simulink model "Model"  (R2018b)
settings: Solver=FixedStepAuto  StartTime=0.0  StopTime=10000  RelTol=1e-3
values from neighbouring files (symbols this model uses):
  Cb = 1000    [workspace.m]
  Ch = 2700    [workspace.m]
  Cw = 4200    [workspace.m]
  Cwym = 2700    [workspace.m]
  Fzcomax = 150    [workspace.m]
  Kext = 15000    [workspace.m]
  Kh = 12000    [workspace.m]
  Kw = 250000    [workspace.m]
  Mb = 20000    [workspace.m]
  Mco = 3000    [workspace.m]
  Mh = 3000    [workspace.m]
  Mm = 3000    [workspace.m]
  ro = 1000    [workspace.m]
  T0 = 5    [workspace.m]
  TrSP = 15    [workspace.m]
libraries: simulink x2
settings Model: Creator=Konrad  LastModifiedBy=Konrad

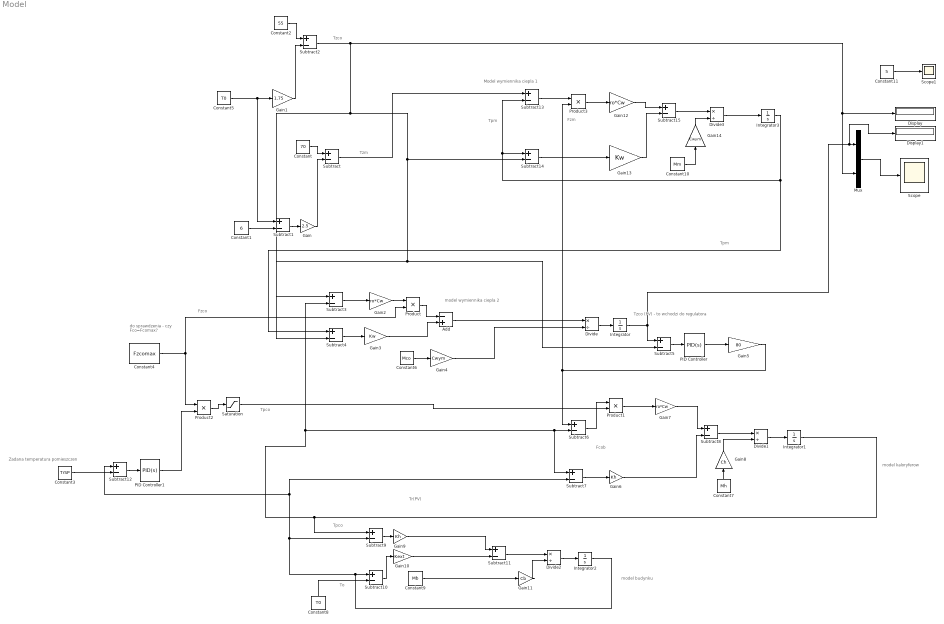
== system Model ==
  note: Model wymiennika ciepla 1
  note: do sprawdzenia
      | - czy Fco=Fcomax?
  note: model budynku
  note: Fcob
  note: Tr(PV)
  note: model kaloryferow
  note: model wymiennika ciepla 2
  note: Tzco (PV) - to wchodzi do regulatora
  note: Fzco
  note: Tpco
  note: Tpm
  note: Tzco
  note: Tzm
  note: Tpco
  note: To
  note: Zadana temperatura pomieszczen
  note: Tpm
  note: Fzm
  Add : Sum  Inputs=-+
  Constant : Constant  Value=70
  Constant1 : Constant  Value=6
  Constant10 : Constant  Value=Mm
  Constant11 : Constant  Value=5
  Constant2 : Constant  Value=55
  Constant3 : Constant  Value=TrSP
  Constant4 : Constant  Value=Fzcomax
  Constant5 : Constant  Value=T0
  Constant6 : Constant  Value=Mco
  Constant7 : Constant  Value=Mh
  Constant8 : Constant  Value=T0
  Constant9 : Constant  Value=Mb
  Display : Display
  Display1 : Display
  Divide{,1..3} (4 alike) : Product  Inputs=*/
  Gain : Gain  Gain=2.5
  Gain1 : Gain  Gain=1.75
  Gain10 : Gain  Gain=Kext
  Gain11 : Gain  Gain=Cb
  Gain12 : Gain  Gain=ro*Cw
  Gain13 : Gain  Gain=Kw
  Gain14 : Gain  Gain=Cwym
  Gain2 : Gain  Gain=ro*Cw
  Gain3 : Gain  Gain=Kw
  Gain4 : Gain  Gain=Cwym
  Gain5 : Gain  Gain=80
  Gain6 : Gain  Gain=Kh
  Gain7 : Gain  Gain=ro*Cw
  Gain8 : Gain  Gain=Ch
  Gain9 : Gain  Gain=Kh
  Integrator{,1..3} (4 alike) : Integrator
  Mux : Mux  Inputs=2
  PID Controller : simulink/Continuous/PID Controller  Controller=PID  Form=Parallel  TimeDomain=Continuous-time  SampleTime=-1  IntegratorMethod=Forward Euler  FilterMethod=Forward Euler  ControllerParametersSource=internal  P=0.01  I=0.1  D=0  UseFilter=on  N=100  TunerSelectOption=Transfer Function Based (PID Tuner App)  InitialConditionSource=internal  InitialConditionForIntegrator=0  InitialConditionForFilter=0  DifferentiatorICPrevScaledInput=0  ExternalReset=none  TrackingMode=off  Kt=1  LimitOutput=on  UpperSaturationLimit=1  LowerSaturationLimit=0  LinearizeAsGain=on  AntiWindupMode=none  Kb=1  POutMin=[]  POutMax=[]  IOutMin=[]  IOutMax=[]  DOutMin=[]  DOutMax=[]  NOutMin=[]  NOutMax=[]  SumOutMin=[]  SumOutMax=[]  SaturationOutMin=[]  SaturationOutMax=[]  PParamMin=[]  PParamMax=[]  IParamMin=[]  IParamMax=[]  DParamMin=[]  DParamMax=[]  NParamMin=[]  NParamMax=[]  KbParamMin=[]  KbParamMax=[]  KtParamMin=[]  KtParamMax=[]  KbOutMin=[]  KbOutMax=[]  KtOutMin=[]  KtOutMax=[]  IntegratorOutMin=[]  IntegratorOutMax=[]  FilterOutMin=[]  FilterOutMax=[]  SumI1OutMin=[]  SumI1OutMax=[]  SumI2OutMin=[]  SumI2OutMax=[]  SumI3OutMin=[]  SumI3OutMax=[]  SumI4OutMin=[]  SumI4OutMax=[]  SumDOutMin=[]  SumDOutMax=[]  DifferentiatorOutMin=[]  DifferentiatorOutMax=[]  FilterDiffOutCoefMin=[]  FilterDiffOutCoefMax=[]  ReciprocalOutMin=[]  ReciprocalOutMax=[]  SumDenOutMin=[]  SumDenOutMax=[]  SumNumOutMin=[]  SumNumOutMax=[]  DivideOutMin=[]  DivideOutMax=[]  IntegratorContinuousStateAttributes=''  IntegratorStateMustResolveToSignalObject=off  IntegratorRTWStateStorageClass=Auto  FilterContinuousStateAttributes=''  FilterStateMustResolveToSignalObject=off  FilterRTWStateStorageClass=Auto  ParallelPVariant=InternalParameters  IdealPVariant=Disabled  IVariant=InternalParameters  DVariant=InternalParameters  IntegratorVariant=Continuous  SatVariant=Enabled  AWVariant=Passthrough  PCopyVariant=Disabled  TRVariant=Disabled  FdbkBlocksVariant=Forward  IdealPFdbkVariant=Disabled  SatFdbkVariant=Disabled  DerivativeFilterVariant=ContFilter  NVariant=InternalParameters  NCopyVariant=Disabled  FilterICVariant=InternalICsFilter  IntegratorICVariant=InternalICs  ExternalResetVariant=Disabled  TRSumVariant=Passthrough  SumFdbkVariant=Disabled  SumVariant=Sum_PID
  PID Controller1 : simulink/Continuous/PID Controller  Controller=PID  Form=Parallel  TimeDomain=Continuous-time  SampleTime=-1  IntegratorMethod=Forward Euler  FilterMethod=Forward Euler  ControllerParametersSource=internal  P=0.01  I=0.1  D=0  UseFilter=on  N=100  TunerSelectOption=Transfer Function Based (PID Tuner App)  InitialConditionSource=internal  InitialConditionForIntegrator=0  InitialConditionForFilter=0  DifferentiatorICPrevScaledInput=0  ExternalReset=none  TrackingMode=off  Kt=1  LimitOutput=on  UpperSaturationLimit=1  LowerSaturationLimit=0  LinearizeAsGain=on  AntiWindupMode=none  Kb=1  POutMin=[]  POutMax=[]  IOutMin=[]  IOutMax=[]  DOutMin=[]  DOutMax=[]  NOutMin=[]  NOutMax=[]  SumOutMin=[]  SumOutMax=[]  SaturationOutMin=[]  SaturationOutMax=[]  PParamMin=[]  PParamMax=[]  IParamMin=[]  IParamMax=[]  DParamMin=[]  DParamMax=[]  NParamMin=[]  NParamMax=[]  KbParamMin=[]  KbParamMax=[]  KtParamMin=[]  KtParamMax=[]  KbOutMin=[]  KbOutMax=[]  KtOutMin=[]  KtOutMax=[]  IntegratorOutMin=[]  IntegratorOutMax=[]  FilterOutMin=[]  FilterOutMax=[]  SumI1OutMin=[]  SumI1OutMax=[]  SumI2OutMin=[]  SumI2OutMax=[]  SumI3OutMin=[]  SumI3OutMax=[]  SumI4OutMin=[]  SumI4OutMax=[]  SumDOutMin=[]  SumDOutMax=[]  DifferentiatorOutMin=[]  DifferentiatorOutMax=[]  FilterDiffOutCoefMin=[]  FilterDiffOutCoefMax=[]  ReciprocalOutMin=[]  ReciprocalOutMax=[]  SumDenOutMin=[]  SumDenOutMax=[]  SumNumOutMin=[]  SumNumOutMax=[]  DivideOutMin=[]  DivideOutMax=[]  IntegratorContinuousStateAttributes=''  IntegratorStateMustResolveToSignalObject=off  IntegratorRTWStateStorageClass=Auto  FilterContinuousStateAttributes=''  FilterStateMustResolveToSignalObject=off  FilterRTWStateStorageClass=Auto  ParallelPVariant=InternalParameters  IdealPVariant=Disabled  IVariant=InternalParameters  DVariant=InternalParameters  IntegratorVariant=Continuous  SatVariant=Enabled  AWVariant=Passthrough  PCopyVariant=Disabled  TRVariant=Disabled  FdbkBlocksVariant=Forward  IdealPFdbkVariant=Disabled  SatFdbkVariant=Disabled  DerivativeFilterVariant=ContFilter  NVariant=InternalParameters  NCopyVariant=Disabled  FilterICVariant=InternalICsFilter  IntegratorICVariant=InternalICs  ExternalResetVariant=Disabled  TRSumVariant=Passthrough  SumFdbkVariant=Disabled  SumVariant=Sum_PID
  Product{,1..3} (4 alike) : Product
  Saturation : Saturate  UpperLimit=40  LowerLimit=0
  Scope : Scope
  Scope1 : Scope
  Subtract{,1..15} (16 alike) : Sum  Inputs=+-
  wires:
  Constant/1 -> Subtract/1
  Constant5/1 -> Subtract1/1, Gain1/1
  Constant1/1 -> Subtract1/2
  Subtract1/1 -> Gain/1
  Gain/1 -> Subtract/2
  Constant2/1 -> Subtract2/1
  Gain1/1 -> Subtract2/2
  Integrator3/1 -> Subtract4/1, Subtract13/2, Subtract14/1
  Integrator1/1 -> Subtract3/2, Subtract7/1, Subtract6/2, Subtract9/1
  Subtract3/1 -> Gain2/1
  Gain2/1 -> Product/1
  Constant4/1 -> Product/2, Product2/1
  Product/1 -> Add/1
  Subtract4/1 -> Gain3/1
  Gain3/1 -> Add/2
  Add/1 -> Divide/1
  Constant6/1 -> Gain4/1
  Gain4/1 -> Divide/2
  Divide/1 -> Integrator/1
  Integrator/1 -> Subtract5/1, Display1/1, Mux/1
  Subtract5/1 -> PID Controller/1
  PID Controller/1 -> Gain5/1
  Integrator2/1 -> Subtract10/1, Subtract9/2, Subtract7/2, Subtract12/1
  Subtract7/1 -> Gain6/1
  Product1/1 -> Gain7/1
  Subtract6/1 -> Product1/1
  Gain7/1 -> Subtract8/1
  Gain6/1 -> Subtract8/2
  Subtract8/1 -> Divide1/1
  Divide1/1 -> Integrator1/1
  Constant7/1 -> Gain8/1
  Gain8/1 -> Divide1/2
  Constant8/1 -> Subtract10/2
  Subtract9/1 -> Gain9/1
  Gain9/1 -> Subtract11/1
  Gain10/1 -> Subtract11/2
  Subtract10/1 -> Gain10/1
  Subtract11/1 -> Divide2/1
  Gain11/1 -> Divide2/2
  Constant9/1 -> Gain11/1
  Divide2/1 -> Integrator2/1
  Subtract12/1 -> PID Controller1/1
  PID Controller1/1 -> Product2/2
  Product2/1 -> Saturation/1
  Saturation/1 -> Product1/2
  Constant3/1 -> Subtract12/2
  Constant10/1 -> Gain14/1
  Gain5/1 -> Product3/2, Subtract6/1
  Gain14/1 -> Divide3/2
  Product3/1 -> Gain12/1
  Divide3/1 -> Integrator3/1
  Subtract/1 -> Subtract13/1
  Subtract14/1 -> Gain13/1
  Gain12/1 -> Subtract15/1
  Subtract15/1 -> Divide3/1
  Subtract13/1 -> Product3/1
  Gain13/1 -> Subtract15/2
  Subtract2/1 -> Display/1, Mux/2, Subtract14/2, Subtract5/2, Subtract4/2, Subtract3/1
  Constant11/1 -> Scope1/1
  Mux/1 -> Scope/1
